simulink model "diskretno_poredjenje_regulatora1"  (R2015a)
settings: Solver=ode45  StartTime=0.0  StopTime=10.0  RelTol=1e-3
libraries: simulink_extras x2
settings Model: Creator=Korisnik  LastModifiedBy=Korisnik

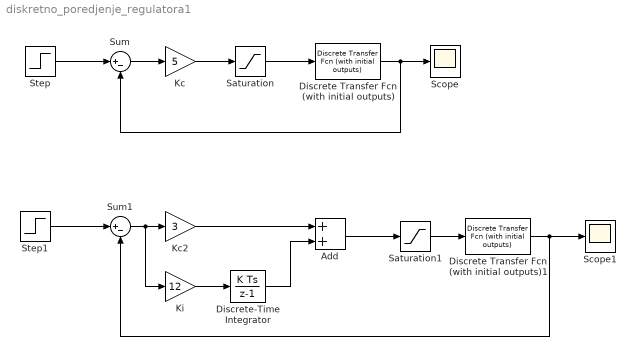
== system diskretno_poredjenje_regulatora1 ==
  Add : Sum
  Discrete Transfer Fcn (with initial outputs) : simulink_extras/Additional Discrete/Discrete Transfer Fcn (with initial outputs)  N=[0.0998613]  D=[1 -0.8751733]  U0=[0]  Y0=0  TS=0.04
  Discrete Transfer Fcn (with initial outputs)1 : simulink_extras/Additional Discrete/Discrete Transfer Fcn (with initial outputs)  N=[0.0998613]  D=[1 -0.8751733]  U0=[0]  Y0=0  TS=0.04
  Discrete-Time Integrator : DiscreteIntegrator  InitialConditionSetting=State (most efficient)  SampleTime=0.04
  Kc : Gain  Gain=5
  Kc2 : Gain  Gain=3
  Ki : Gain  Gain=12
  Saturation : Saturate  UpperLimit=125  LowerLimit=0
  Saturation1 : Saturate  UpperLimit=125  LowerLimit=0
  Scope : Scope
  Scope1 : Scope
  Step : Step  After=100  SampleTime=0
  Step1 : Step  After=100  SampleTime=0
  Sum : Sum  Inputs=|+-
  Sum1 : Sum  Inputs=|+-
  wires:
  Step/1 -> Sum/1
  Sum/1 -> Kc/1
  Kc/1 -> Saturation/1
  Discrete Transfer Fcn (with initial outputs)/1 -> Scope/1, Sum/2
  Step1/1 -> Sum1/1
  Sum1/1 -> Ki/1, Kc2/1
  Add/1 -> Saturation1/1
  Kc2/1 -> Add/1
  Discrete Transfer Fcn (with initial outputs)1/1 -> Sum1/2, Scope1/1
  Ki/1 -> Discrete-Time Integrator/1
  Discrete-Time Integrator/1 -> Add/2
  Saturation/1 -> Discrete Transfer Fcn (with initial outputs)/1
  Saturation1/1 -> Discrete Transfer Fcn (with initial outputs)1/1
